simulink model "mmc_model"  (R2023b)
settings: Solver=VariableStepAuto  StartTime=0.0  StopTime=simulation.tsim  RelTol=1e-3
values from neighbouring files (symbols this model uses):
  ab0_to_cell = inv(cell_to_2ab0)    [init_mmc.m]
  cell_to_2ab0 = kron(abc_to_ab0, abc_to_ab0)    [init_mmc.m]
  grid_to_cell = kron(eye(3), ones(3, 1))    [init_mmc.m]
  J = [0 -1; 1 0]    [init_mmc.m]
  machine_to_cell = kron(ones(3, 1), eye(3))    [init_mmc.m]
  volt_to_cell = [      [          1 0 0 0 0 0 ... (first row only)    [init_mmc.m]
undefined symbols (not defined in the file or in its folder): avi, clc, cpu, ctrl, currentControl, DiscIntNeverNeededParam, gfl, grid, load2, loadStep, machine, mmc, pq_ctrl, simulation, soa, stiffGrid, sync, testScenario
libraries: library x17, spsThreePhaseSeriesRLCBranchLib x16, eeGeneralControl x15, spsControlledVoltageSourceLib x15, simulink x11, spsThreePhaseVIMeasurementLib x10, spsGroundLib x9, eeDiscretePi x8, simulink_extras x8, spsabctodq0Lib x8, spsThreePhaseBreakerLib x7, spsdq0toabcLib x5
(part 3 of 3)

== system mmc_model/Electrical Model/Variant Subsystem/GFL_VSC/Measurements ==
  wt : Inport
  v_abc : Inport  Port=2
  i_abc : Inport  Port=3
  abc_dq_1 : spsabctodq0Lib/abc to dq0  Alignment=Aligned with phase A axis
  abc_dq_3 : spsabctodq0Lib/abc to dq0  Alignment=Aligned with phase A axis
  v_dq : Outport
  i_dq : Outport  Port=2
  wires:
  v_abc/1 -> abc_dq_1/1
  abc_dq_1/1 -> v_dq/1
  abc_dq_3/1 -> i_dq/1
  wt/1 -> abc_dq_3/2, abc_dq_1/2
  i_abc/1 -> abc_dq_3/1

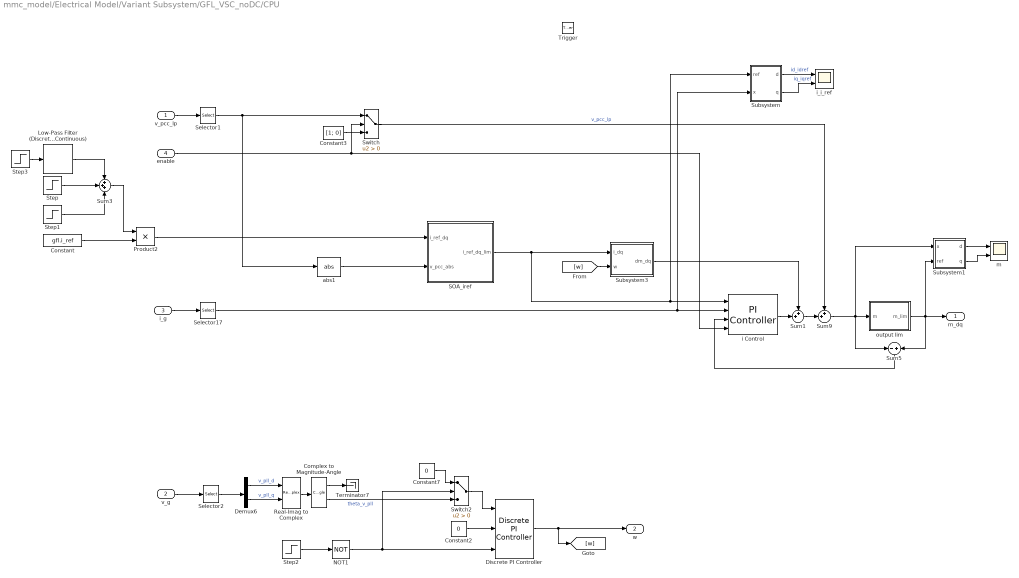
== system mmc_model/Electrical Model/Variant Subsystem/GFL_VSC_noDC/CPU ==
  v_pcc_lp : Inport
  v_g : Inport  Port=2
  i_g : Inport  Port=3
  enable : Inport  Port=4
  Trigger : TriggerPort  VariantControl=(inherit)
  Complex to Magnitude-Angle : ComplexToMagnitudeAngle
  Constant : Constant  Value=gfl.i_ref
  Constant2 : Constant  Value=0
  Constant3 : Constant  Value=[1; 0]
  Constant7 : Constant  Value=0
  Demux6 : Demux  Outputs=2
  Discrete PI Controller : eeDiscretePi/Discrete PI Controller  Kp=ctrl.machine.pll.kp  Ki=ctrl.machine.pll.ti  Kaw=1  x0=ctrl.machine.pll.w0  Ts=-1
      settings: LibrarySourceBlock=ee_sl_lib/General Control/Discrete PI Controller
  Low-Pass Filter (Discrete or Continuous) : eeGeneralControl/Low-Pass Filter (Discrete or Continuous)  K=1  T=1e-1  B=inf  A=-inf  init_option=Inherited from block input  x0=0  Ts=-1
  NOT1 : Logic  Operator=NOT  IconShape=distinctive  AllPortsSameDT=off  OutDataTypeStr=boolean
  Product2 : Product
  Real-Imag to Complex : RealImagToComplex
  SOA_iref : Subsystem
  Selector1 : Selector  InputPortWidth=3  IndexOptions=Index vector (dialog)  Indices=[1 2]  OutputSizes=1
  Selector17 : Selector  InputPortWidth=3  IndexOptions=Index vector (dialog)  Indices=[1 2]  OutputSizes=1
  Selector2 : Selector  InputPortWidth=3  IndexOptions=Index vector (dialog)  Indices=[1 2]  OutputSizes=1
  Step : Step  Time=loadStep.stepDown  After=-1
  Step1 : Step  Time=loadStep.stepUp
  Step2 : Step  Time=gfl.pll_enable
  Step3 : Step  Time=gfl.ref_step
  Subsystem : Subsystem
  Subsystem1 : Subsystem
  Subsystem3 : Subsystem
  Sum1 : Sum  Inputs=++|
  Sum3 : Sum  Inputs=+++
  Sum5 : Sum  Inputs=-|+
  Sum9 : Sum  Inputs=++|
  Switch : Switch  Criteria=u2 > Threshold  SaturateOnIntegerOverflow=off  InputSameDT=off
  Switch2 : Switch  Criteria=u2 > Threshold  SaturateOnIntegerOverflow=off  InputSameDT=off
  Terminator7 : Terminator
  abs1 : library/abs  SystemSampleTime=-1  VariantActivationTime=update diagram  AllowFlexibleInterface=on  Latency=0  AutoFrameSizeCalculation=off
  i Control : library/PI Controller  VariantControl=overcurr_ctrl.sel==1  kp=ctrl.machine.ictrl.kp  ti=ctrl.machine.ictrl.ti  Kaw=1000
  i_i_ref : Scope  NumInputPorts=2
  m : Scope  NumInputPorts=2
  output lim : Subsystem
  m_dq : Outport
  w : Outport  Port=2
  wires:
  i_g/1 -> Selector17/1
  Switch/1 -> Sum9/1  "v_pcc_lp"
  Sum1/1 -> Sum9/2
  enable/1 -> i Control/4, Switch/2
  Sum9/1 -> output lim/1(m), Sum5/1, Subsystem1/1(x)
  [w] -> Subsystem3/2(w)
  v_pcc_lp/1 -> Selector1/1
  Constant3/1 -> Switch/3
  Sum5/1 -> i Control/3
  Subsystem/1(d) -> i_i_ref/1  "id_idref"
  Subsystem/2(q) -> i_i_ref/2  "iq_iqref"
  Subsystem1/2(q) -> m/2
  Subsystem1/1(d) -> m/1
  Step3/1 -> Low-Pass Filter (Discrete or Continuous)/1
  Subsystem3/1(dm_dq) -> Sum1/1
  output lim/1(m_lim) -> Subsystem1/2(ref), m_dq/1, Sum5/2
  i Control/1 -> Sum1/2
  Selector17/1 -> Subsystem/2(x), i Control/2
  Selector1/1 -> abs1/1, Switch/1
  Constant2/1 -> Discrete PI Controller/2
  Discrete PI Controller/1 -> [w], w/1
  NOT1/1 -> Switch2/2, Discrete PI Controller/3
  Real-Imag to Complex/1 -> Complex to Magnitude-Angle/1
  Constant7/1 -> Switch2/1
  Step2/1 -> NOT1/1
  Complex to Magnitude-Angle/2 -> Switch2/3  "theta_v_pll"
  Demux6/2 -> Real-Imag to Complex/2  "v_pll_q"
  Complex to Magnitude-Angle/1 -> Terminator7/1
  Demux6/1 -> Real-Imag to Complex/1  "v_pll_d"
  Switch2/1 -> Discrete PI Controller/1
  v_g/1 -> Selector2/1
  Selector2/1 -> Demux6/1
  SOA_iref/1(i_ref_dq_lim) -> Subsystem/1(ref), i Control/1, Subsystem3/1(i_dq)
  abs1/1 -> SOA_iref/2(v_pcc_abs)
  Step/1 -> Sum3/2
  Low-Pass Filter (Discrete or Continuous)/1 -> Sum3/1
  Step1/1 -> Sum3/3
  Product2/1 -> SOA_iref/1(i_ref_dq)
  Sum3/1 -> Product2/1
  Constant/1 -> Product2/2

== system mmc_model/Electrical Model/Variant Subsystem/GFL_VSC_noDC/Measurements ==
  wt : Inport
  v_abc : Inport  Port=2
  i_abc : Inport  Port=3
  abc_dq_1 : spsabctodq0Lib/abc to dq0  Alignment=Aligned with phase A axis
  abc_dq_3 : spsabctodq0Lib/abc to dq0  Alignment=Aligned with phase A axis
  v_dq : Outport
  i_dq : Outport  Port=2
  wires:
  v_abc/1 -> abc_dq_1/1
  abc_dq_1/1 -> v_dq/1
  abc_dq_3/1 -> i_dq/1
  wt/1 -> abc_dq_3/2, abc_dq_1/2
  i_abc/1 -> abc_dq_3/1

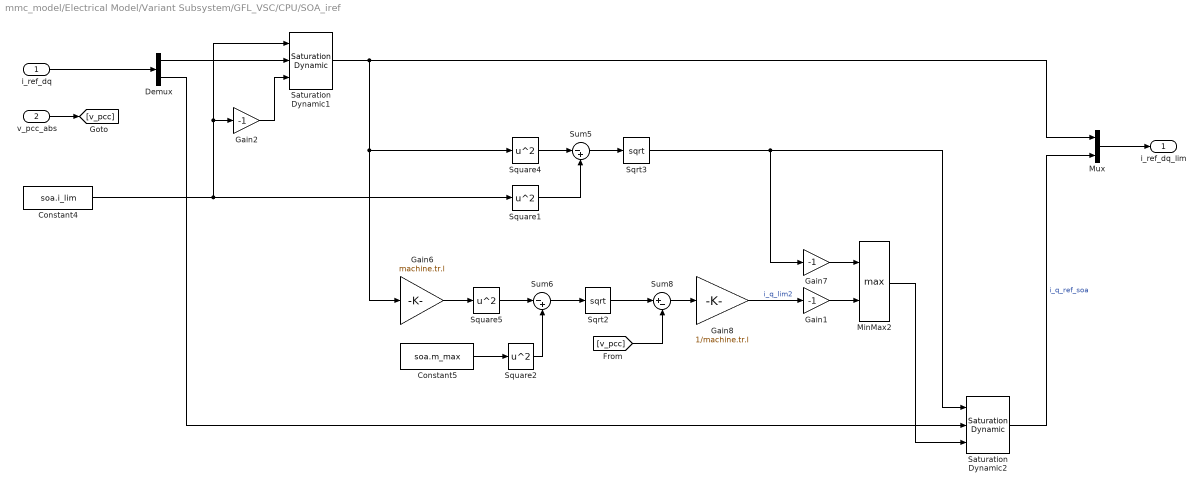
== system mmc_model/Electrical Model/Variant Subsystem/GFL_VSC/CPU/SOA_iref ==
  i_ref_dq : Inport
  v_pcc_abs : Inport  Port=2
  Constant4 : Constant  Value=soa.i_lim
  Constant5 : Constant  Value=soa.m_max
  Demux : Demux  Outputs=2
  Gain1 : Gain  Gain=-1
  Gain2 : Gain  Gain=-1
  Gain6 : Gain  Gain=machine.tr.l
  Gain7 : Gain  Gain=-1
  Gain8 : Gain  Gain=1/machine.tr.l
  MinMax2 : MinMax  Function=max  Inputs=2
  Mux : Mux  Inputs=2
  Saturation Dynamic1 : simulink/Discontinuities/Saturation Dynamic  OutMin=[]  OutMax=[]  OutDataTypeStr=Inherit: Same as second input  OutDataType=fixdt(1, 16)  OutScaling=2^-10  DoSatur=off
  Saturation Dynamic2 : simulink/Discontinuities/Saturation Dynamic  OutMin=[]  OutMax=[]  OutDataTypeStr=Inherit: Same as second input  OutDataType=fixdt(1, 16)  OutScaling=2^-10  DoSatur=off
  Sqrt2 : Sqrt
  Sqrt3 : Sqrt
  Square{1..2,4..5} (4 alike) : Math  Operator=square
  Sum5 : Sum  Inputs=|-+
  Sum6 : Sum  Inputs=|-+
  Sum8 : Sum  Inputs=|+-
  i_ref_dq_lim : Outport
  wires:
  Saturation Dynamic1/1 -> Square4/1, Gain6/1, Mux/1
  Gain8/1 -> Gain1/1  "i_q_lim2"
  Sqrt3/1 -> Gain7/1, Saturation Dynamic2/1
  Gain6/1 -> Square5/1
  Demux/1 -> Saturation Dynamic1/2
  Square4/1 -> Sum5/1
  Square5/1 -> Sum6/1
  Sum8/1 -> Gain8/1
  Sum5/1 -> Sqrt3/1
  Demux/2 -> Saturation Dynamic2/2
  Constant4/1 -> Saturation Dynamic1/1, Gain2/1, Square1/1
  MinMax2/1 -> Saturation Dynamic2/3
  i_ref_dq/1 -> Demux/1
  Gain7/1 -> MinMax2/1
  Sum6/1 -> Sqrt2/1
  Saturation Dynamic2/1 -> Mux/2  "i_q_ref_soa"
  Mux/1 -> i_ref_dq_lim/1
  Gain1/1 -> MinMax2/2
  v_pcc_abs/1 -> [v_pcc]
  Sqrt2/1 -> Sum8/1
  [v_pcc] -> Sum8/2
  Square1/1 -> Sum5/2
  Gain2/1 -> Saturation Dynamic1/3
  Square2/1 -> Sum6/2
  Constant5/1 -> Square2/1

== system mmc_model/Electrical Model/Variant Subsystem/GFL_VSC/CPU/Subsystem ==
  ref : Inport
  x : Inport  Port=2
  Demux : Demux  Outputs=2
  Demux1 : Demux  Outputs=2
  Mux1 : Mux  Inputs=2
  Mux2 : Mux  Inputs=2
  d : Outport
  q : Outport  Port=2
  wires:
  Mux2/1 -> q/1
  x/1 -> Demux1/1
  Demux/2 -> Mux2/1
  Demux1/2 -> Mux2/2
  Demux/1 -> Mux1/1
  Demux1/1 -> Mux1/2
  Mux1/1 -> d/1
  ref/1 -> Demux/1

== system mmc_model/Electrical Model/Variant Subsystem/GFL_VSC/CPU/Subsystem1 ==
  x : Inport
  ref : Inport  Port=2
  Demux : Demux  Outputs=2
  Demux1 : Demux  Outputs=2
  Mux1 : Mux  Inputs=2
  Mux2 : Mux  Inputs=2
  d : Outport
  q : Outport  Port=2
  wires:
  Mux2/1 -> q/1
  ref/1 -> Demux1/1
  Demux/2 -> Mux2/1
  Demux1/2 -> Mux2/2
  Demux/1 -> Mux1/1
  Demux1/1 -> Mux1/2
  Mux1/1 -> d/1
  x/1 -> Demux/1

== system mmc_model/Electrical Model/Variant Subsystem/GFL_VSC/CPU/Subsystem3 ==
  i_dq : Inport
  w : Inport  Port=2
  Gain : Gain  Gain=J  Multiplication=Matrix(K*u) (u vector)
  Gain1 : Gain  Gain=machine.tr.l
  Gain2 : Gain  Gain=machine.tr.r
  Product : Product
  Sum8 : Sum  Inputs=++|
  dm_dq : Outport
  wires:
  Gain1/1 -> Sum8/2
  Sum8/1 -> dm_dq/1  "dm_dq"
  Product/1 -> Gain/1
  Gain/1 -> Gain1/1  "dm_dq"
  w/1 -> Product/1
  i_dq/1 -> Gain2/1, Product/2
  Gain2/1 -> Sum8/1

== system mmc_model/Electrical Model/Variant Subsystem/GFL_VSC/CPU/output lim ==
  m : Inport
  Cartesian to Polar : simulink_extras/Transformations/Cartesian to Polar
  Constant1 : Constant  Value=soa.m_max
  Demux6 : Demux  Outputs=2
  MinMax2 : MinMax  Inputs=2
  Mux : Mux  Inputs=2
  Polar to Cartesian : simulink_extras/Transformations/Polar to Cartesian
  m_lim : Outport
  wires:
  Polar to Cartesian/2 -> Mux/2
  MinMax2/1 -> Polar to Cartesian/1
  Constant1/1 -> MinMax2/1
  Cartesian to Polar/2 -> Polar to Cartesian/2
  Demux6/1 -> Cartesian to Polar/1
  Polar to Cartesian/1 -> Mux/1
  Demux6/2 -> Cartesian to Polar/2
  Cartesian to Polar/1 -> MinMax2/2
  Mux/1 -> m_lim/1
  m/1 -> Demux6/1

== system mmc_model/Electrical Model/Variant Subsystem/GFL_VSC_noDC/CPU/SOA_iref ==
  i_ref_dq : Inport
  v_pcc_abs : Inport  Port=2
  Constant4 : Constant  Value=soa.i_lim
  Constant5 : Constant  Value=soa.m_max
  Demux : Demux  Outputs=2
  Gain1 : Gain  Gain=-1
  Gain2 : Gain  Gain=-1
  Gain6 : Gain  Gain=machine.tr.l
  Gain7 : Gain  Gain=-1
  Gain8 : Gain  Gain=1/machine.tr.l
  MinMax2 : MinMax  Function=max  Inputs=2
  Mux : Mux  Inputs=2
  Saturation Dynamic1 : simulink/Discontinuities/Saturation Dynamic  OutMin=[]  OutMax=[]  OutDataTypeStr=Inherit: Same as second input  OutDataType=fixdt(1, 16)  OutScaling=2^-10  DoSatur=off
  Saturation Dynamic2 : simulink/Discontinuities/Saturation Dynamic  OutMin=[]  OutMax=[]  OutDataTypeStr=Inherit: Same as second input  OutDataType=fixdt(1, 16)  OutScaling=2^-10  DoSatur=off
  Sqrt2 : Sqrt
  Sqrt3 : Sqrt
  Square{1..2,4..5} (4 alike) : Math  Operator=square
  Sum5 : Sum  Inputs=|-+
  Sum6 : Sum  Inputs=|-+
  Sum8 : Sum  Inputs=|+-
  i_ref_dq_lim : Outport
  wires:
  Saturation Dynamic1/1 -> Square4/1, Gain6/1, Mux/1
  Gain8/1 -> Gain1/1  "i_q_lim2"
  Sqrt3/1 -> Gain7/1, Saturation Dynamic2/1
  Gain6/1 -> Square5/1
  Demux/1 -> Saturation Dynamic1/2
  Square4/1 -> Sum5/1
  Square5/1 -> Sum6/1
  Sum8/1 -> Gain8/1
  Sum5/1 -> Sqrt3/1
  Demux/2 -> Saturation Dynamic2/2
  Constant4/1 -> Saturation Dynamic1/1, Gain2/1, Square1/1
  MinMax2/1 -> Saturation Dynamic2/3
  i_ref_dq/1 -> Demux/1
  Gain7/1 -> MinMax2/1
  Sum6/1 -> Sqrt2/1
  Saturation Dynamic2/1 -> Mux/2  "i_q_ref_soa"
  Mux/1 -> i_ref_dq_lim/1
  Gain1/1 -> MinMax2/2
  v_pcc_abs/1 -> [v_pcc]
  Sqrt2/1 -> Sum8/1
  [v_pcc] -> Sum8/2
  Square1/1 -> Sum5/2
  Gain2/1 -> Saturation Dynamic1/3
  Square2/1 -> Sum6/2
  Constant5/1 -> Square2/1

== system mmc_model/Electrical Model/Variant Subsystem/GFL_VSC_noDC/CPU/Subsystem ==
  ref : Inport
  x : Inport  Port=2
  Demux : Demux  Outputs=2
  Demux1 : Demux  Outputs=2
  Mux1 : Mux  Inputs=2
  Mux2 : Mux  Inputs=2
  d : Outport
  q : Outport  Port=2
  wires:
  Mux2/1 -> q/1
  x/1 -> Demux1/1
  Demux/2 -> Mux2/1
  Demux1/2 -> Mux2/2
  Demux/1 -> Mux1/1
  Demux1/1 -> Mux1/2
  Mux1/1 -> d/1
  ref/1 -> Demux/1

== system mmc_model/Electrical Model/Variant Subsystem/GFL_VSC_noDC/CPU/Subsystem1 ==
  x : Inport
  ref : Inport  Port=2
  Demux : Demux  Outputs=2
  Demux1 : Demux  Outputs=2
  Mux1 : Mux  Inputs=2
  Mux2 : Mux  Inputs=2
  d : Outport
  q : Outport  Port=2
  wires:
  Mux2/1 -> q/1
  ref/1 -> Demux1/1
  Demux/2 -> Mux2/1
  Demux1/2 -> Mux2/2
  Demux/1 -> Mux1/1
  Demux1/1 -> Mux1/2
  Mux1/1 -> d/1
  x/1 -> Demux/1

== system mmc_model/Electrical Model/Variant Subsystem/GFL_VSC_noDC/CPU/Subsystem3 ==
  i_dq : Inport
  w : Inport  Port=2
  Gain : Gain  Gain=J  Multiplication=Matrix(K*u) (u vector)
  Gain1 : Gain  Gain=machine.tr.l
  Gain2 : Gain  Gain=machine.tr.r
  Product : Product
  Sum8 : Sum  Inputs=++|
  dm_dq : Outport
  wires:
  Gain1/1 -> Sum8/2
  Sum8/1 -> dm_dq/1  "dm_dq"
  Product/1 -> Gain/1
  Gain/1 -> Gain1/1  "dm_dq"
  w/1 -> Product/1
  i_dq/1 -> Gain2/1, Product/2
  Gain2/1 -> Sum8/1

== system mmc_model/Electrical Model/Variant Subsystem/GFL_VSC_noDC/CPU/output lim ==
  m : Inport
  Cartesian to Polar : simulink_extras/Transformations/Cartesian to Polar
  Constant1 : Constant  Value=soa.m_max
  Demux6 : Demux  Outputs=2
  MinMax2 : MinMax  Inputs=2
  Mux : Mux  Inputs=2
  Polar to Cartesian : simulink_extras/Transformations/Polar to Cartesian
  m_lim : Outport
  wires:
  Polar to Cartesian/2 -> Mux/2
  MinMax2/1 -> Polar to Cartesian/1
  Constant1/1 -> MinMax2/1
  Cartesian to Polar/2 -> Polar to Cartesian/2
  Demux6/1 -> Cartesian to Polar/1
  Polar to Cartesian/1 -> Mux/1
  Demux6/2 -> Cartesian to Polar/2
  Cartesian to Polar/1 -> MinMax2/2
  Mux/1 -> m_lim/1
  m/1 -> Demux6/1

== matlab function mmc_model/CPU/Current Limiting Control/Safety Filter/MATLAB Function ==
  data: u input; dm output; dm_corr output; lambda output
function [dm, dm_corr, lambda] = fcn(u)
    
    % safety.f_data = [-23.561944901923447,376.99111843077515,0.0,0.0,0.0,0.0,0.0;-376.99111843077515,-23.561944901923447,0.0,0.0,0.0,0.0,0.0;0.0,0.0,-100.0,0.0,0.0,0.0,0.0;0.0,0.0,0.0,-100.0,0.0,0.0,0.0;0.0,0.0,0.0,0.0,0.0,0.0,0.0;0.0,0.0,0.0,0.0,0.0,0.0,0.0;0.0,0.0,0.0,0.0,0.0,0.0,0.0];
    % safety.G_data = [2356.194490192345;0.0;0.0;0.0;0.0;0.0;0.0;0.0;2356.194490192345;0.0;0.0;0.0;0.0;0.0];
    % safety.V_data = [-1.0000000000137432,-9.608728963220513e-10,-3.1526780939938525e-10,-4.008540187830507e-09,-1.4998587508899322e-08,1.155827152569663e-09,3.5810538888140883e-10,1.5873015872814367,4.699027810611526,-3.5222976609873145e-07,-6.990257033176867,-15.145906374976814,-4.575859599942044,-0.012277507962152271,-8.652943174571386e-07,-3.5222976609873145e-07,4.699026905933879,15.145899840237334,-6.990247940034223,0.012278293915240393,-4.5758595909229065,-1.223007625673093e-08,-6.990257033176867,15.145899840237334,115.4755112639637,1.1898166744934225e-06,7.863557723819616,-16.834855979709577,-6.888762156608453e-06,-15.145906374976814,-6.990247940034223,1.1898166744934225e-06,115.4754749401915,16.834872640837578,7.863543143719876,-1.14106375719361e-05,-4.575859599942044,0.012278293915240393,7.863557723819616,16.834872640837578,5.146405637511074,-4.307100795325092e-07,1.0353412927011278e-06,-0.012277507962152271,-4.5758595909229065,-16.834855979709577,7.863543143719876,-4.307100795325092e-07,5.146406868745372,-1.4251828594785418e-09,-8.652943174571386e-07,-1.223007625673093e-08,-6.888762156608453e-06,-1.14106375719361e-05,1.0353412927011278e-06,-1.4251828594785418e-09,-0.6298815447469528];
    % safety.B_data = [-1.0,-1.271349346743454e-13,-4.728046188242939e-14,-1.3618001279042881e-14,-3.759532202585598e-14,-2.2042619773147842e-14,1.3448680318419533e-13,1.587301587277223,0.6298815931096612,-3.0315926153871147e-12,-1.0994365101753219e-11,-4.6565682469944224e-11,-1.2398042837095638e-08,3.6863640853951274e-12,-1.1895185308030092e-13,-3.0315926153871147e-12,0.6298815930955556,4.7257973936971416e-11,-1.2014901576377734e-11,3.420260273916765e-12,-1.2382159672818403e-08,9.50088233361252e-14,-1.0994365101753219e-11,4.7257973936971416e-11,2.4966040533824684e-08,-5.436857987617307e-12,-1.0174559832792565e-11,3.953625170439576e-11,-4.986971821394681e-14,-4.6565682469944224e-11,-1.2014901576377734e-11,-5.436857987617307e-12,2.4962256101305552e-08,-4.023269423388052e-11,-9.079761187389751e-12,-9.171198202407077e-15,-1.2398042837095638e-08,3.420260273916765e-12,-1.0174559832792565e-11,-4.023269423388052e-11,1.4114769262374208e-08,-4.1616791912714206e-12,8.698689969993056e-14,3.6863640853951274e-12,-1.2382159672818403e-08,3.953625170439576e-11,-9.079761187389751e-12,-4.1616791912714206e-12,1.4096895463731896e-08,-1.0106454442471979e-13,-1.1895185308030092e-13,9.50088233361252e-14,-4.986971821394681e-14,-9.171198202407077e-15,8.698689969993056e-14,-1.0106454442471979e-13,-0.6298815697536329];
    % safety.nV_data = [-9.608728963220513e-10,9.398055621223053,-7.044595321974629e-07,-13.980514066353734,-30.29181274995363,-9.151719199884088,-0.024555015924304542,-1.7305886349142773e-06;-3.1526780939938525e-10,-7.044595321974629e-07,9.398053811867758,30.291799680474668,-13.980495880068446,0.024556587830480786,-9.151719181845813,-2.446015251346186e-08;-4.008540187830507e-09,-13.980514066353734,30.291799680474668,230.9510225279274,2.379633348986845e-06,15.727115447639232,-33.66971195941915,-1.3777524313216906e-05;-1.4998587508899322e-08,-30.29181274995363,-13.980495880068446,2.379633348986845e-06,230.950949880383,33.669745281675155,15.727086287439752,-2.28212751438722e-05;1.155827152569663e-09,-9.151719199884088,0.024556587830480786,15.727115447639232,33.669745281675155,10.292811275022148,-8.614201590650184e-07,2.0706825854022557e-06;3.5810538888140883e-10,-0.024555015924304542,-9.151719181845813,-33.66971195941915,15.727086287439752,-8.614201590650184e-07,10.292813737490745,-2.8503657189570836e-09;1.5873015872814367,-1.7305886349142773e-06,-2.446015251346186e-08,-1.3777524313216906e-05,-2.28212751438722e-05,2.0706825854022557e-06,-2.8503657189570836e-09,-1.2597630894939056];
    % safety.nB_data = [-1.271349346743454e-13,1.2597631862193224,-6.063185230774229e-12,-2.1988730203506438e-11,-9.313136493988845e-11,-2.4796085674191275e-08,7.372728170790255e-12,-2.3790370616060183e-13;-4.728046188242939e-14,-6.063185230774229e-12,1.2597631861911112,9.451594787394283e-11,-2.402980315275547e-11,6.84052054783353e-12,-2.4764319345636805e-08,1.900176466722504e-13;-1.3618001279042881e-14,-2.1988730203506438e-11,9.451594787394283e-11,4.993208106764937e-08,-1.0873715975234615e-11,-2.034911966558513e-11,7.907250340879152e-11,-9.973943642789362e-14;-3.759532202585598e-14,-9.313136493988845e-11,-2.402980315275547e-11,-1.0873715975234615e-11,4.9924512202611104e-08,-8.046538846776104e-11,-1.8159522374779503e-11,-1.8342396404814155e-14;-2.2042619773147842e-14,-2.4796085674191275e-08,6.84052054783353e-12,-2.034911966558513e-11,-8.046538846776104e-11,2.8229538524748416e-08,-8.323358382542841e-12,1.7397379939986112e-13;1.3448680318419533e-13,7.372728170790255e-12,-2.4764319345636805e-08,7.907250340879152e-11,-1.8159522374779503e-11,-8.323358382542841e-12,2.819379092746379e-08,-2.0212908884943957e-13;1.587301587277223,-2.3790370616060183e-13,1.900176466722504e-13,-9.973943642789362e-14,-1.8342396404814155e-14,1.7397379939986112e-13,-2.0212908884943957e-13,-1.2597631395072657];
    % safety.gamma_V_data = [210.92427255435327];
    % safety.gamma_B_data = [683.37013935184709];

    % safety.f_data = [-23.56,376.99,0.0,0.0,0.0,0.0,0.0;-376.99,-23.56,0.0,0.0,0.0,0.0,0.0;0.0,0.0,-100.0,0.0,0.0,0.0,0.0;0.0,0.0,0.0,-100.0,0.0,0.0,0.0;0.0,0.0,0.0,0.0,0.0,0.0,0.0;0.0,0.0,0.0,0.0,0.0,0.0,0.0;0.0,0.0,0.0,0.0,0.0,0.0,0.0];
    % safety.G_data = [2356.19;0.0;0.0;0.0;0.0;0.0;0.0;0.0;2356.19;0.0;0.0;0.0;0.0;0.0];
    % safety.V_data = [-1.0,-0.0,-0.0,-0.0,-0.0,0.0,0.0,1.59,4.7,-0.0,-6.99,-15.15,-4.58,-0.01,-0.0,-0.0,4.7,15.15,-6.99,0.01,-4.58,-0.0,-6.99,15.15,115.48,0.0,7.86,-16.83,-0.0,-15.15,-6.99,0.0,115.48,16.83,7.86,-0.0,-4.58,0.01,7.86,16.83,5.15,-0.0,0.0,-0.01,-4.58,-16.83,7.86,-0.0,5.15,-0.0,-0.0,-0.0,-0.0,-0.0,0.0,-0.0,-0.63];
    % safety.B_data = [-1.0,-0.0,-0.0,-0.0,-0.0,-0.0,0.0,1.59,0.63,-0.0,-0.0,-0.0,-0.0,0.0,-0.0,-0.0,0.63,0.0,-0.0,0.0,-0.0,0.0,-0.0,0.0,0.0,-0.0,-0.0,0.0,-0.0,-0.0,-0.0,-0.0,0.0,-0.0,-0.0,-0.0,-0.0,0.0,-0.0,-0.0,0.0,-0.0,0.0,0.0,-0.0,0.0,-0.0,-0.0,0.0,-0.0,-0.0,0.0,-0.0,-0.0,0.0,-0.0,-0.63];
    % safety.nV_data = [-0.0,9.4,-0.0,-13.98,-30.29,-9.15,-0.02,-0.0;-0.0,-0.0,9.4,30.29,-13.98,0.02,-9.15,-0.0;-0.0,-13.98,30.29,230.95,0.0,15.73,-33.67,-0.0;-0.0,-30.29,-13.98,0.0,230.95,33.67,15.73,-0.0;0.0,-9.15,0.02,15.73,33.67,10.29,-0.0,0.0;0.0,-0.02,-9.15,-33.67,15.73,-0.0,10.29,-0.0;1.59,-0.0,-0.0,-0.0,-0.0,0.0,-0.0,-1.26];
    % safety.nB_data = [-0.0,1.26,-0.0,-0.0,-0.0,-0.0,0.0,-0.0;-0.0,-0.0,1.26,0.0,-0.0,0.0,-0.0,0.0;-0.0,-0.0,0.0,0.0,-0.0,-0.0,0.0,-0.0;-0.0,-0.0,-0.0,-0.0,0.0,-0.0,-0.0,-0.0;-0.0,-0.0,0.0,-0.0,-0.0,0.0,-0.0,0.0;0.0,0.0,-0.0,0.0,-0.0,-0.0,0.0,-0.0;1.59,-0.0,0.0,-0.0,-0.0,0.0,-0.0,-1.26];
    % safety.gamma_V_data = [210.92427255435327];
    % safety.gamma_B_data = [683.37013935184709];
    
    safety.f_data = [-23.56,376.99,0.0,0.0,0.0,0.0,0.0;-376.99,-23.56,0.0,0.0,0.0,0.0,0.0;0.0,0.0,-100.0,0.0,0.0,0.0,0.0;0.0,0.0,0.0,-100.0,0.0,0.0,0.0;0.0,0.0,0.0,0.0,0.0,0.0,0.0;0.0,0.0,0.0,0.0,0.0,0.0,0.0;0.0,0.0,0.0,0.0,0.0,0.0,0.0];
    safety.G_data = [2356.19;0.0;0.0;0.0;0.0;0.0;0.0;0.0;2356.19;0.0;0.0;0.0;0.0;0.0];
    safety.V_data = [-1.0,0.0,0.0,-0.0,0.0,-0.0,-0.0,1.59,4.44,0.0,-7.34,-16.01,-4.32,-0.01,-0.0,0.0,4.44,16.01,-7.34,0.01,-4.32,0.0,-7.34,16.01,109.67,-0.0,8.36,-18.05,-0.0,-16.01,-7.34,-0.0,109.67,18.05,8.36,-0.0,-4.32,0.01,8.36,18.05,4.89,0.0,0.0,-0.01,-4.32,-18.05,8.36,0.0,4.89,-0.0,-0.0,0.0,-0.0,-0.0,0.0,-0.0,-0.63];
    safety.B_data = [-1.0,-0.0,-0.0,-0.0,-0.0,0.0,0.0,1.59,0.63,0.0,-0.0,-0.0,-0.0,-0.0,0.0,0.0,0.63,0.0,-0.0,-0.0,-0.0,0.0,-0.0,0.0,0.0,0.0,0.0,0.0,-0.0,-0.0,-0.0,0.0,0.0,0.0,0.0,-0.0,-0.0,-0.0,0.0,0.0,0.0,0.0,-0.0,-0.0,-0.0,0.0,0.0,0.0,0.0,-0.0,0.0,0.0,-0.0,-0.0,-0.0,-0.0,-0.63];
    safety.nV_data = [0.0,8.89,0.0,-14.68,-32.01,-8.64,-0.02,-0.0;0.0,0.0,8.89,32.01,-14.68,0.02,-8.64,0.0;-0.0,-14.68,32.01,219.34,-0.0,16.72,-36.09,-0.0;0.0,-32.01,-14.68,-0.0,219.34,36.09,16.72,-0.0;-0.0,-8.64,0.02,16.72,36.09,9.78,0.0,0.0;-0.0,-0.02,-8.64,-36.09,16.72,0.0,9.78,-0.0;1.59,-0.0,0.0,-0.0,-0.0,0.0,-0.0,-1.26];
    safety.nB_data = [-0.0,1.26,0.0,-0.0,-0.0,-0.0,-0.0,0.0;-0.0,0.0,1.26,0.0,-0.0,-0.0,-0.0,0.0;-0.0,-0.0,0.0,0.0,0.0,0.0,0.0,-0.0;-0.0,-0.0,-0.0,0.0,0.0,0.0,0.0,-0.0;0.0,-0.0,-0.0,0.0,0.0,0.0,0.0,-0.0;0.0,-0.0,-0.0,0.0,0.0,0.0,0.0,-0.0;1.59,0.0,0.0,-0.0,-0.0,-0.0,-0.0,-1.26];
    safety.gamma_V_data = [206.71];
    safety.gamma_B_data = [2820.01];

    % safety.f_data = [-23.56,376.99,0.0,0.0,0.0,0.0,0.0;-376.99,-23.56,0.0,0.0,0.0,0.0,0.0;0.0,0.0,-100.0,0.0,0.0,0.0,0.0;0.0,0.0,0.0,-100.0,0.0,0.0,0.0;0.0,0.0,0.0,0.0,0.0,0.0,0.0;0.0,0.0,0.0,0.0,0.0,0.0,0.0;0.0,0.0,0.0,0.0,0.0,0.0,0.0];
    % safety.G_data = [2356.19;0.0;0.0;0.0;0.0;0.0;0.0;0.0;2356.19;0.0;0.0;0.0;0.0;0.0];
    % safety.V_data = [-1.0,-0.0,0.0,-0.0,0.0,0.0,-0.0,1.59,4.58,-0.0,-7.14,-15.5,-4.45,-0.01,-0.0,-0.0,4.58,15.5,-7.14,0.01,-4.45,0.0,-7.14,15.5,112.51,-0.0,8.08,-17.35,-0.0,-15.5,-7.14,-0.0,112.51,17.35,8.08,-0.0,-4.45,0.01,8.08,17.35,5.02,-0.0,0.0,-0.01,-4.45,-17.35,8.08,-0.0,5.02,-0.0,-0.0,0.0,-0.0,-0.0,0.0,-0.0,-0.63];
    % safety.B_data = [-1.0,-0.0,-0.0,0.0,0.0,0.0,0.0,1.59,0.63,-0.0,-0.0,-0.0,-0.0,0.0,-0.0,-0.0,0.63,0.0,0.0,0.0,-0.0,0.0,-0.0,0.0,0.0,0.0,0.0,-0.0,-0.0,-0.0,0.0,0.0,0.0,0.0,-0.0,-0.0,-0.0,0.0,0.0,0.0,0.0,-0.0,0.0,0.0,-0.0,-0.0,-0.0,-0.0,0.0,-0.0,-0.0,0.0,-0.0,-0.0,0.0,-0.0,-0.63];
    % safety.nV_data = [-0.0,9.15,-0.0,-14.29,-31.01,-8.9,-0.02,-0.0;0.0,-0.0,9.15,31.01,-14.29,0.02,-8.9,0.0;-0.0,-14.29,31.01,225.02,-0.0,16.17,-34.7,-0.0;0.0,-31.01,-14.29,-0.0,225.02,34.7,16.17,-0.0;0.0,-8.9,0.02,16.17,34.7,10.04,-0.0,0.0;-0.0,-0.02,-8.9,-34.7,16.17,-0.0,10.04,-0.0;1.59,-0.0,0.0,-0.0,-0.0,0.0,-0.0,-1.26];
    % safety.nB_data = [-0.0,1.26,-0.0,-0.0,-0.0,-0.0,0.0,-0.0;-0.0,-0.0,1.26,0.0,0.0,0.0,-0.0,0.0;0.0,-0.0,0.0,0.0,0.0,0.0,-0.0,-0.0;0.0,-0.0,0.0,0.0,0.0,0.0,-0.0,-0.0;0.0,-0.0,0.0,0.0,0.0,0.0,-0.0,0.0;0.0,0.0,-0.0,-0.0,-0.0,-0.0,0.0,-0.0;1.59,-0.0,0.0,-0.0,-0.0,0.0,-0.0,-1.26];
    % safety.gamma_V_data = [108.96];
    % safety.gamma_B_data = [192.09];

    cpu.ts = 200e-6;

    % read input arguments
    dm_ref = u(1:2);
    i_ref = u(3:4);
    i = u(5:6);
    dv_pcc = u(7:8);
    enable = u(9);
    i0 = u(10);

    if ~enable

        dm = dm_ref;

        dm_corr = [0; 0];
        lambda = [0; 0];

        return

    end

    x = [i; dv_pcc; i_ref; i0];

    xx = reshape(x * x', [], 1);

    x01 = [1;x];
    x02 = [1;xx];
    x012 = [1;x;xx];

    V = safety.V_data * x012;
    B = safety.B_data * x012;

    u_ref = dm_ref + dv_pcc;

    f_sys = safety.f_data * x;
    G_sys = reshape(safety.G_data, 7, 2);

    nV = safety.nV_data * x01;
    nB = safety.nB_data * x01;

    gamma_V = safety.gamma_V_data;
    gamma_B = safety.gamma_B_data;

    % cost = (1/2) * x' * H * x + f' * x
    H = eye(2);
    f = -u_ref;

    % A x <= b
    A = [ ...
           nB' * G_sys;
           nV' * G_sys ...
        ];       
    b = [ ...
           -nB' * f_sys - gamma_B * B;
           -nV' * f_sys - gamma_V * V ...
         ];

    lb = [-2; -2];
    ub = [2; 2];

    x0 = u_ref;

    options = optimoptions('quadprog', 'Algorithm', 'active-set');
    [u, ~, ~, ~, lambda_val] = quadprog(H, f, A, b, [], [], lb, ub, x0, options);

    % update states
    dm = u - dv_pcc;

    % debugging
    dm_corr = u - u_ref;
    lambda = lambda_val.ineqlin;

== matlab function mmc_model/CPU/Current Limiting Control/Safety Filter B only/MATLAB Function ==
  data: u input; dm output; dm_corr output; lambda output
function [dm, dm_corr, lambda] = fcn(u)

    % safety.f_data = [-23.56,376.99,0.0,0.0,0.0,0.0,0.0;-376.99,-23.56,0.0,0.0,0.0,0.0,0.0;0.0,0.0,-100.0,0.0,0.0,0.0,0.0;0.0,0.0,0.0,-100.0,0.0,0.0,0.0;0.0,0.0,0.0,0.0,0.0,0.0,0.0;0.0,0.0,0.0,0.0,0.0,0.0,0.0;0.0,0.0,0.0,0.0,0.0,0.0,0.0];
    % safety.G_data = [2356.19;0.0;0.0;0.0;0.0;0.0;0.0;0.0;2356.19;0.0;0.0;0.0;0.0;0.0];
    % safety.V_data = [-1.0,-0.0,-0.0,-0.0,-0.0,0.0,0.0,1.59,4.7,-0.0,-6.99,-15.15,-4.58,-0.01,-0.0,-0.0,4.7,15.15,-6.99,0.01,-4.58,-0.0,-6.99,15.15,115.48,0.0,7.86,-16.83,-0.0,-15.15,-6.99,0.0,115.48,16.83,7.86,-0.0,-4.58,0.01,7.86,16.83,5.15,-0.0,0.0,-0.01,-4.58,-16.83,7.86,-0.0,5.15,-0.0,-0.0,-0.0,-0.0,-0.0,0.0,-0.0,-0.63];
    % safety.B_data = [-1.0,-0.0,-0.0,-0.0,-0.0,-0.0,0.0,1.59,0.63,-0.0,-0.0,-0.0,-0.0,0.0,-0.0,-0.0,0.63,0.0,-0.0,0.0,-0.0,0.0,-0.0,0.0,0.0,-0.0,-0.0,0.0,-0.0,-0.0,-0.0,-0.0,0.0,-0.0,-0.0,-0.0,-0.0,0.0,-0.0,-0.0,0.0,-0.0,0.0,0.0,-0.0,0.0,-0.0,-0.0,0.0,-0.0,-0.0,0.0,-0.0,-0.0,0.0,-0.0,-0.63];
    % safety.nV_data = [-0.0,9.4,-0.0,-13.98,-30.29,-9.15,-0.02,-0.0;-0.0,-0.0,9.4,30.29,-13.98,0.02,-9.15,-0.0;-0.0,-13.98,30.29,230.95,0.0,15.73,-33.67,-0.0;-0.0,-30.29,-13.98,0.0,230.95,33.67,15.73,-0.0;0.0,-9.15,0.02,15.73,33.67,10.29,-0.0,0.0;0.0,-0.02,-9.15,-33.67,15.73,-0.0,10.29,-0.0;1.59,-0.0,-0.0,-0.0,-0.0,0.0,-0.0,-1.26];
    % safety.nB_data = [-0.0,1.26,-0.0,-0.0,-0.0,-0.0,0.0,-0.0;-0.0,-0.0,1.26,0.0,-0.0,0.0,-0.0,0.0;-0.0,-0.0,0.0,0.0,-0.0,-0.0,0.0,-0.0;-0.0,-0.0,-0.0,-0.0,0.0,-0.0,-0.0,-0.0;-0.0,-0.0,0.0,-0.0,-0.0,0.0,-0.0,0.0;0.0,0.0,-0.0,0.0,-0.0,-0.0,0.0,-0.0;1.59,-0.0,0.0,-0.0,-0.0,0.0,-0.0,-1.26];
    % safety.gamma_V_data = [210.92427255435327];
    % safety.gamma_B_data = [683.37013935184709];

    safety.f_data = [-23.56,376.99,0.0,0.0,0.0,0.0,0.0;-376.99,-23.56,0.0,0.0,0.0,0.0,0.0;0.0,0.0,-100.0,0.0,0.0,0.0,0.0;0.0,0.0,0.0,-100.0,0.0,0.0,0.0;0.0,0.0,0.0,0.0,0.0,0.0,0.0;0.0,0.0,0.0,0.0,0.0,0.0,0.0;0.0,0.0,0.0,0.0,0.0,0.0,0.0];
    safety.G_data = [2356.19;0.0;0.0;0.0;0.0;0.0;0.0;0.0;2356.19;0.0;0.0;0.0;0.0;0.0];
    safety.V_data = [-1.0,0.0,0.0,-0.0,0.0,-0.0,-0.0,1.59,4.44,0.0,-7.34,-16.01,-4.32,-0.01,-0.0,0.0,4.44,16.01,-7.34,0.01,-4.32,0.0,-7.34,16.01,109.67,-0.0,8.36,-18.05,-0.0,-16.01,-7.34,-0.0,109.67,18.05,8.36,-0.0,-4.32,0.01,8.36,18.05,4.89,0.0,0.0,-0.01,-4.32,-18.05,8.36,0.0,4.89,-0.0,-0.0,0.0,-0.0,-0.0,0.0,-0.0,-0.63];
    safety.B_data = [-1.0,-0.0,-0.0,-0.0,-0.0,0.0,0.0,1.59,0.63,0.0,-0.0,-0.0,-0.0,-0.0,0.0,0.0,0.63,0.0,-0.0,-0.0,-0.0,0.0,-0.0,0.0,0.0,0.0,0.0,0.0,-0.0,-0.0,-0.0,0.0,0.0,0.0,0.0,-0.0,-0.0,-0.0,0.0,0.0,0.0,0.0,-0.0,-0.0,-0.0,0.0,0.0,0.0,0.0,-0.0,0.0,0.0,-0.0,-0.0,-0.0,-0.0,-0.63];
    safety.nV_data = [0.0,8.89,0.0,-14.68,-32.01,-8.64,-0.02,-0.0;0.0,0.0,8.89,32.01,-14.68,0.02,-8.64,0.0;-0.0,-14.68,32.01,219.34,-0.0,16.72,-36.09,-0.0;0.0,-32.01,-14.68,-0.0,219.34,36.09,16.72,-0.0;-0.0,-8.64,0.02,16.72,36.09,9.78,0.0,0.0;-0.0,-0.02,-8.64,-36.09,16.72,0.0,9.78,-0.0;1.59,-0.0,0.0,-0.0,-0.0,0.0,-0.0,-1.26];
    safety.nB_data = [-0.0,1.26,0.0,-0.0,-0.0,-0.0,-0.0,0.0;-0.0,0.0,1.26,0.0,-0.0,-0.0,-0.0,0.0;-0.0,-0.0,0.0,0.0,0.0,0.0,0.0,-0.0;-0.0,-0.0,-0.0,0.0,0.0,0.0,0.0,-0.0;0.0,-0.0,-0.0,0.0,0.0,0.0,0.0,-0.0;0.0,-0.0,-0.0,0.0,0.0,0.0,0.0,-0.0;1.59,0.0,0.0,-0.0,-0.0,-0.0,-0.0,-1.26];
    safety.gamma_V_data = [206.71];
    safety.gamma_B_data = [2820.01];

    cpu.ts = 200e-6;

    % read input arguments
    dm_ref = u(1:2);
    i_ref = u(3:4);
    i = u(5:6);
    dv_pcc = u(7:8);
    enable = u(9);
    i0 = u(10);

    if ~enable

        dm = dm_ref;

        dm_corr = [0; 0];
        lambda = [0; 0];

        return

    end
        
    x = [i; dv_pcc; i_ref; i0];

    xx = reshape(x * x', [], 1);

    x01 = [1;x];
    x012 = [1;x;xx];

    B = safety.B_data * x012;

    u_ref = dm_ref + dv_pcc;

    f_sys = safety.f_data * x;
    G_sys = reshape(safety.G_data, 7, 2);

    nB = safety.nB_data * x01;

    gamma_B = safety.gamma_B_data;

    % cost = (1/2) * x' * H * x + f' * x
    H = eye(2);
    f = -u_ref;

    % A x <= b
    A = nB' * G_sys;       
    b = -nB' * f_sys - gamma_B * B;

    lb = [-2; -2];
    ub = [2; 2];

    x0 = u_ref;

    options = optimoptions('quadprog', 'Algorithm', 'active-set');
    [u, ~, ~, ~, lambda_val] = quadprog(H, f, A, b, [], [], lb, ub, x0, options);

    % update states
    dm = u - dv_pcc;

    % debugging
    dm_corr = u - u_ref;
    lambda = [lambda_val.ineqlin; 0];
